simulink model "sedemo_discouragearrival"  (Simulink 7.5)
settings: Solver=VariableStepDiscrete  StartTime=0.0  StopTime=100000  MaxStep=inf  RelTol=1e-3
PostLoadFcn:
  | open_system([gcs '/Service Rate Gain']);
  | open_system([gcs '/Waiting Time Comparison:  Theory vs. Simulation']);
undefined symbols (not defined in the file or in its folder): des_subsystemblock, des_subsysteminport, des_subsystemoutport, des_subsystemsupportblock
libraries: simulink x2, simeventstranslate1 x2, simeventssink1 x1, simeventsqueue1 x1, simeventsinfo x1, simeventsserver1 x1, simeventsgenerators1 x1
CloseFcn:
  | close_system([gcs '/Service Rate Gain']);
  | close_system([gcs '/Waiting Time Comparison:  Theory vs. Simulation']);
settings Model: Creator=The MathWorks Inc.  ExtModeAutoUpdateStatusClock=off
settings DataIOCC: SaveOutput=off  SaveTime=off
settings OptimizationCC: InlineInvariantSignals=on  InitFltsAndDblsToZero=on  BufferReusableBoundary=off
settings DebuggingCC: AlgebraicLoopMsg=error  SaveWithParameterizedLinksMsg=none  SignalResolutionControl=TryResolveAllWithWarning  SolverPrmCheckMsg=none  MultiTaskDSMMsg=warning  MultiTaskCondExecSysMsg=none  SigSpecEnsureSampleTimeMsg=none  BusObjectLabelMismatch=none  StrictBusMsg=None
settings RTWCC: IncludeERTFirstTime=on
settings GRTTargetCC: TargetFcnLib=ansi_tfl_tmw.mat
settings SimEventsCC: propIdentEventSeed=12345678  propDiagAttribOutput=1  propDiagFcnCallOutput=1  propDiagStatOutput=0

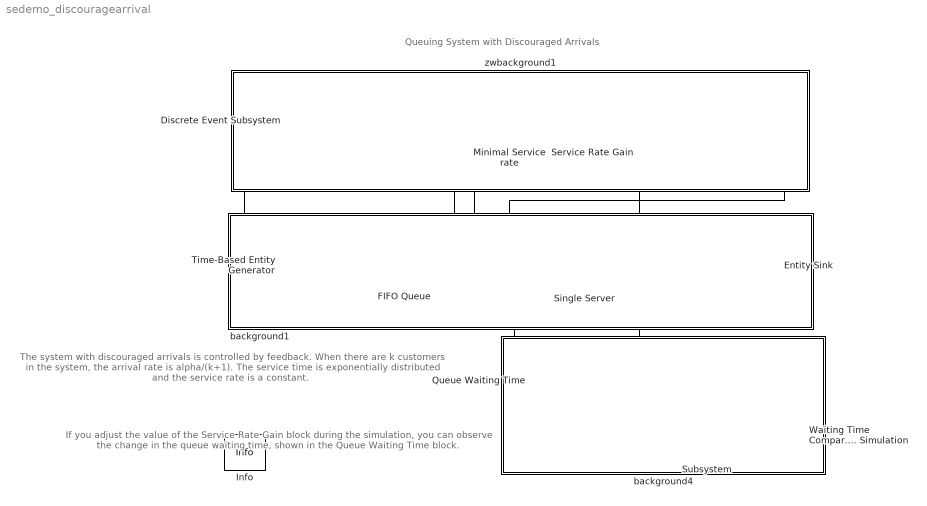
== system sedemo_discouragearrival ==
  note: Queuing System with Discouraged Arrivals
  note: The system with discouraged arrivals is
      | controlled by feedback. When there are k
      | customers in the system, the arrival rate is
      | alpha/(k+1). The service time is exponentially
      | distributed and the service rate is a constant.
  note: If you adjust the value of the Service Rate
      | Gain block during the simulation, you
      | can observe the change in the queue waiting
      | time, shown in the Queue Waiting Time block.
  "  " : Subsystem  mask(Exponential Service Time Distribution){seed=1234567}
      mask prompts: seed "Initial seed"
      mask help: For a given input service rate, output an exponentially distributed random number. Output is repeatable for a given seed.
      mask Display: disp('Exponential\nService Time\nDistribution');
  Discrete Event Subsystem : Subsystem  LoadFcn=des_subsystemblock(gcb, 'load');  InitFcn=des_subsystemblock(gcb, 'init');  StartFcn=des_subsystemblock(gcb, 'start');  StopFcn=des_subsystemblock(gcb, 'stop');  mask(Discrete Event Subsystem){seed=9876543}
      mask prompts: seed "Initial seed:"
      settings: CopyFcn=des_subsystemblock(gcb, 'copy');  DeleteFcn=des_subsystemblock(gcb, 'delete');  UndoDeleteFcn=des_subsystemblock(gcb, 'undodelete');  ModelCloseFcn=des_subsystemblock(gcb, 'modelclose');  PreSaveFcn=des_subsystemblock(gcb, 'presave');  NameChangeFcn=des_subsystemblock(gcb, 'namechange');  OpenFcn=des_subsystemblock(gcb, 'open');  ParentCloseFcn=des_subsystemblock(gcb, 'parentclose');  ErrorFcn=des_subsystemerror
      mask Help: helpview(simeventsbhelp);
      mask Display: disp('Interarrival Time Distribution\n with Discouraged Rate\n(Alpha=1)');
  Entity Sink : simeventssink1/Entity Sink  Priority=1  SystemSampleTime=-1  AvailableForArrivals=on  StatNumberArrived=Off
  FIFO Queue : simeventsqueue1/FIFO Queue  Priority=1  SystemSampleTime=-1  Capacity=Inf  EnableTOPort=off  StatNumberDeparted=Off  StatNumberInBlock=On  StatPendingEntity=Off  StatAverageWait=On  StatAverageQueueLength=Off  StatNumberTimedout=Off
  Info : simeventsinfo/Info  SystemSampleTime=-1
  Minimal Service rate : Constant  OutDataType=sfix(16)  OutScaling=2^0
  Queue Waiting Time : Display
  Service Rate Gain : simulink/Math Operations/Slider Gain  SystemSampleTime=-1  low=0.1  gain=3  high=10
  Single Server : simeventsserver1/Single Server  Priority=1  SystemSampleTime=-1  ServiceTimeFrom=Signal port t  ServiceTime=1  AttributeName=ServiceTime  PriorityServiceCompletion=1  PermitPreemption=off  SortingAttributeName=PriorityAttributeName  SortingDirection=Ascending  WriteToAttribute=off  ResidualAttributeName=ResidualServiceTime  CreateAttribute=on  EnableTOPort=off  StatNumberDeparted=Off  StatNumberInBlock=On  StatNumberPreempted=Off  StatPendingEntity=Off  StatAverageWait=Off  StatUtilization=Off  StatNumberTimedout=Off
  Subsystem : Subsystem
      mask Type: Waiting Time Evaluation for Discouraged Arrivals
      mask Description: For a given input service rate and alpha=1, evaluate waiting time for discouraged arrivals. Combine and output the theoretical and simulation results.
      mask Display: disp('Waiting Time\nEvaluation');
  Time-Based Entity Generator : simeventsgenerators1/Entity Generators/Time-Based Entity Generator  Priority=1  DialogController=des_ddg_create  DialogControllerArgs=DataTag13  SystemSampleTime=-1  GenerateEntitiesUpon=Intergeneration time from port t  Distribution=Constant  Minimum=0  Maximum=1  Mean=1  InitialSeed=12345  Period=1  PriorityEntityGeneration=1  GenerateEntityAtSimulationStart=on  ResponseWhenBlocked=Pause generation  ResponseWhenUnblocked=Immediate restart  EntityType=Standard  StatNumberDeparted=Off  StatPendingEntity=Off  StatAverageIntergenerationTime=Off
  Waiting Time Comparison:  Theory vs. Simulation : Scope
      settings: YMin=0  YMax=0.15
  background1 : Subsystem
      mask Display: disp('')
  background4 : Subsystem
      mask Display: disp('')
  zwbackground1 : Subsystem
      mask Display: disp('')
  wires:
  "  "/1(Out1) -> Single Server/1
  Discrete Event Subsystem/1(Dout) -> Time-Based Entity Generator/1
  Single Server/1 -> Discrete Event Subsystem/1(Din)
  Minimal Service rate/1 -> Service Rate Gain/1
  Service Rate Gain/1 -> "  "/1(Service rate), Subsystem/1(mu)
  Subsystem/1(Out1) -> Waiting Time Comparison:  Theory vs. Simulation/1
  FIFO Queue/1 -> Discrete Event Subsystem/2(Din1)
  FIFO Queue/2 -> Queue Waiting Time/1, Subsystem/2(waiting time measurement)
  connections:
  Time-Based Entity Generator/RConn1 -- FIFO Queue/LConn1
  FIFO Queue/RConn1 -- Single Server/LConn1
  Single Server/RConn1 -- Entity Sink/LConn1

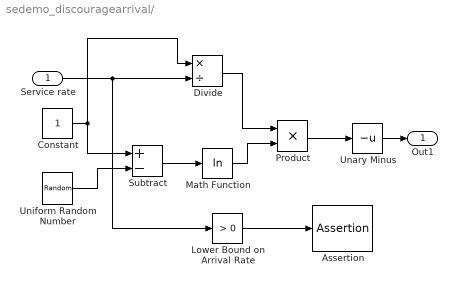
== system sedemo_discouragearrival/   ==
  Service rate : Inport  OutDataType=sfix(16)  OutScaling=2^0
  Assertion : Assertion  Enabled=on
  Constant : Constant  OutDataType=sfix(16)  OutScaling=2^0
  Divide : Product  Inputs=*/  OutDataType=sfix(16)  OutScaling=2^-10
  Lower Bound on Arrival Rate : simulink/Logic and Bit Operations/Compare To Constant  SystemSampleTime=-1  relop=>  const=0  LogicOutDataTypeMode=uint8  ZeroCross=off
  Math Function : Math  Operator=log  OutDataType=sfix(16)  OutScaling=2^0  SaturateOnIntegerOverflow=on
  Product : Product  OutDataType=sfix(16)  OutScaling=2^0  RndMeth=Zero
  Subtract : Sum  Inputs=+-  OutDataType=sfix(16)  OutScaling=2^-10
  Unary Minus : UnaryMinus
  Uniform Random Number : UniformRandomNumber  Minimum=0  Seed=seed  SampleTime=0
  Out1 : Outport  OutDataType=sfix(16)  OutScaling=2^0
  wires:
  Unary Minus/1 -> Out1/1
  Product/1 -> Unary Minus/1
  Math Function/1 -> Product/2
  Subtract/1 -> Math Function/1
  Uniform Random Number/1 -> Subtract/2
  Constant/1 -> Subtract/1, Divide/1
  Service rate/1 -> Divide/2, Lower Bound on Arrival Rate/1
  Divide/1 -> Product/1
  Lower Bound on Arrival Rate/1 -> Assertion/1

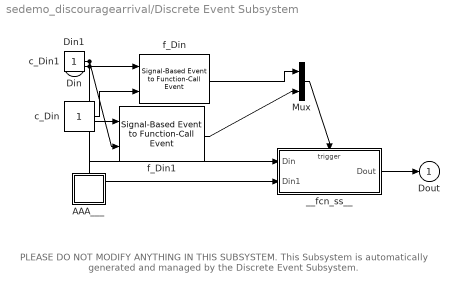
== system sedemo_discouragearrival/Discrete Event Subsystem ==
  note: PLEASE DO NOT MODIFY ANYTHING IN THIS SUBSYSTEM.
      | This Subsystem is automatically generated and
      | managed by the Discrete Event Subsystem.
  Din : Inport  PortDimensions=1  DataType=double  OutDataType=sfix(16)  OutScaling=2^0  OutDataTypeStr=double
  Din1 : Inport  Port=2  PortDimensions=1  DataType=double  OutDataType=sfix(16)  OutScaling=2^0  OutDataTypeStr=double
  AAA___ : Subsystem  LoadFcn=des_subsystemsupportblock(gcb, 'load');  InitFcn=des_subsystemsupportblock(gcb, 'init');  StartFcn=des_subsystemsupportblock(gcb, 'start');  StopFcn=des_subsystemsupportblock(gcb, 'stop');
      settings: CopyFcn=des_subsystemsupportblock(gcb, 'copy');  DeleteFcn=des_subsystemsupportblock(gcb, 'delete');  UndoDeleteFcn=des_subsystemsupportblock(gcb, 'undodelete');  ModelCloseFcn=des_subsystemsupportblock(gcb, 'modelclose');  PreSaveFcn=des_subsystemsupportblock(gcb, 'presave');  NameChangeFcn=des_subsystemsupportblock(gcb, 'namechange');  OpenFcn=des_subsystemsupportblock(gcb, 'open');  ParentCloseFcn=des_subsystemsupportblock(gcb, 'parentclose');
  Mux : Mux  Inputs=2
  __fcn_ss__ : Subsystem  TreatAsAtomicUnit=on
      settings: PropExecContextOutsideSubsystem=on
  c_Din : Constant  OutDataType=sfix(16)  OutScaling=2^0
  c_Din1 : Constant  OutDataType=sfix(16)  OutScaling=2^0
  f_Din : simeventstranslate1/Signal-Based Event to Function-Call Event  Priority=1  SystemSampleTime=-1  GenerateFunctionCallUpon=Sample time hit from port ts  SignalEdgeOption=Rising  EnableE1Port=on  EnableF2Port=off  EnableE2Port=off  SpecifyEventPriority=off  PriorityFunctionCall=20  FunctionCallDelayFrom=Dialog  DelayFunctionCall=0  StatNumberF1Calls=Off  StatNumberF2Calls=Off  MaskBlockType=none
  f_Din1 : simeventstranslate1/Signal-Based Event to Function-Call Event  Priority=1  SystemSampleTime=-1  GenerateFunctionCallUpon=Sample time hit from port ts  SignalEdgeOption=Rising  EnableE1Port=on  EnableF2Port=off  EnableE2Port=off  SpecifyEventPriority=off  PriorityFunctionCall=20  FunctionCallDelayFrom=Dialog  DelayFunctionCall=0  StatNumberF1Calls=Off  StatNumberF2Calls=Off  MaskBlockType=none
  Dout : Outport  OutDataType=sfix(16)  OutScaling=2^0
  wires:
  __fcn_ss__/1(Dout) -> Dout/1
  f_Din/1 -> Mux/1
  c_Din/1 -> f_Din/2
  Mux/1 -> __fcn_ss__/Trigger
  f_Din1/1 -> Mux/2
  c_Din1/1 -> f_Din1/2
  Din/1 -> f_Din/1, __fcn_ss__/1(Din)
  Din1/1 -> f_Din1/1, __fcn_ss__/2(Din1)

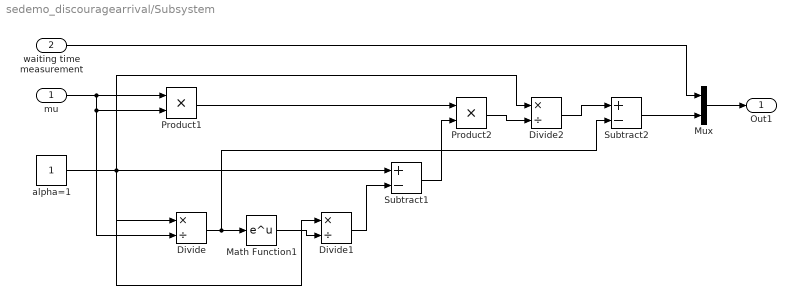
== system sedemo_discouragearrival/Subsystem ==
  mu : Inport  OutDataType=sfix(16)  OutScaling=2^0
  waiting time measurement : Inport  Port=2  OutDataType=sfix(16)  OutScaling=2^0
  Divide : Product  Inputs=*/  OutDataType=sfix(16)  OutScaling=2^-10
  Divide1 : Product  Inputs=*/  OutDataType=sfix(16)  OutScaling=2^-10
  Divide2 : Product  Inputs=*/  OutDataType=sfix(16)  OutScaling=2^-10
  Math Function1 : Math  OutDataType=sfix(16)  OutScaling=2^0  SaturateOnIntegerOverflow=on
  Mux : Mux  Inputs=2
  Product1 : Product  OutDataType=sfix(16)  OutScaling=2^0  RndMeth=Zero
  Product2 : Product  OutDataType=sfix(16)  OutScaling=2^0  RndMeth=Zero
  Subtract1 : Sum  Inputs=+-  OutDataType=sfix(16)  OutScaling=2^-10
  Subtract2 : Sum  Inputs=+-  OutDataType=sfix(16)  OutScaling=2^-10
  alpha=1 : Constant  OutDataType=sfix(16)  OutScaling=2^0
  Out1 : Outport  OutDataType=sfix(16)  OutScaling=2^0
  wires:
  mu/1 -> Divide/2, Product1/2, Product1/1
  alpha=1/1 -> Subtract1/1, Divide/1, Divide1/1, Divide2/1
  Divide/1 -> Math Function1/1, Subtract2/2
  Math Function1/1 -> Divide1/2
  Divide1/1 -> Subtract1/2
  Product1/1 -> Product2/1
  Subtract1/1 -> Product2/2
  Product2/1 -> Divide2/2
  waiting time measurement/1 -> Mux/1
  Mux/1 -> Out1/1
  Divide2/1 -> Subtract2/1
  Subtract2/1 -> Mux/2

== system sedemo_discouragearrival/background1 ==

== system sedemo_discouragearrival/background4 ==

== system sedemo_discouragearrival/zwbackground1 ==
  note: This subsystem is empty

== system sedemo_discouragearrival/Discrete Event Subsystem/AAA___ ==

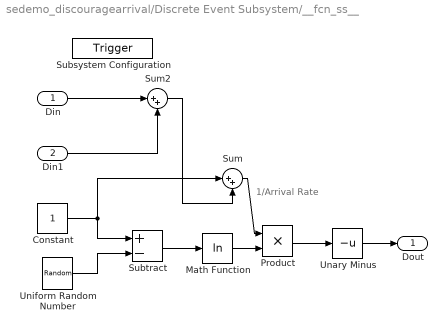
== system sedemo_discouragearrival/Discrete Event Subsystem/__fcn_ss__ ==
  note: 1/Arrival Rate
  Din : Inport  LoadFcn=des_subsysteminport(gcb, 'load');  InitFcn=des_subsysteminport(gcb, 'init');  StartFcn=des_subsysteminport(gcb, 'start');  StopFcn=des_subsysteminport(gcb, 'stop');  OutDataType=sfix(16)  OutScaling=2^0  mask(Discrete Event Inport){PermitSubsystemEvents=on, TypeOfEvent=Sample time hit, SignalEdgeOption=Rising, SpecifyEventPriority=off, PrioritySubsystemEvent=20}
      mask prompts: PermitSubsystemEvents "Execute subsystem upon signal-based events"; TypeOfEvent "Type of signal-based event:"; SignalEdgeOption "Type of change in signal value:"; SpecifyEventPriority "Specify event priority for executing subsystem"; PrioritySubsystemEvent "Subsystem execution event priority:"
      mask help: Input port for a Discrete Event Subsystem block. This block can conditionally execute the subsystem upon signal-based events that meet specified criteria.
      mask init:
      | des_subsystemmask(gcb, 'init','apply')
      settings: CopyFcn=des_subsysteminport(gcb, 'copy');  DeleteFcn=des_subsysteminport(gcb, 'delete');  UndoDeleteFcn=des_subsysteminport(gcb, 'undodelete');  ModelCloseFcn=des_subsysteminport(gcb, 'modelclose');  PreSaveFcn=des_subsysteminport(gcb, 'presave');  NameChangeFcn=des_subsysteminport(gcb, 'namechange');  ParentCloseFcn=des_subsysteminport(gcb, 'parentclose');
      mask Help: helpview(simeventsbhelp);
      mask StyleString: checkbox,popup(Change in signal|Trigger|Sample time hit),popup(Rising|Falling|Either),checkbox,edit
      mask CallbackString: des_subsystemmask(gcb, 'cbPermitSubsystemEvents', 'noapply');|des_subsystemmask(gcb,'cbTypeOfEvent','noapply');||des_subsystemmask(gcb, 'cbSpecifyEventPriority', 'noapply');|
  Din1 : Inport  LoadFcn=des_subsysteminport(gcb, 'load');  InitFcn=des_subsysteminport(gcb, 'init');  StartFcn=des_subsysteminport(gcb, 'start');  StopFcn=des_subsysteminport(gcb, 'stop');  Port=2  OutDataType=sfix(16)  OutScaling=2^0  mask(Discrete Event Inport){PermitSubsystemEvents=on, TypeOfEvent=Sample time hit, SignalEdgeOption=Rising, SpecifyEventPriority=off, PrioritySubsystemEvent=20}
      mask prompts: PermitSubsystemEvents "Execute subsystem upon signal-based events"; TypeOfEvent "Type of signal-based event:"; SignalEdgeOption "Type of change in signal value:"; SpecifyEventPriority "Specify event priority for executing subsystem"; PrioritySubsystemEvent "Subsystem execution event priority:"
      mask help: Input port for a Discrete Event Subsystem block. This block can conditionally execute the subsystem upon signal-based events that meet specified criteria.
      mask init:
      | des_subsystemmask(gcb, 'init','apply')
      settings: CopyFcn=des_subsysteminport(gcb, 'copy');  DeleteFcn=des_subsysteminport(gcb, 'delete');  UndoDeleteFcn=des_subsysteminport(gcb, 'undodelete');  ModelCloseFcn=des_subsysteminport(gcb, 'modelclose');  PreSaveFcn=des_subsysteminport(gcb, 'presave');  NameChangeFcn=des_subsysteminport(gcb, 'namechange');  ParentCloseFcn=des_subsysteminport(gcb, 'parentclose');
      mask Help: helpview(simeventsbhelp);
      mask StyleString: checkbox,popup(Change in signal|Trigger|Sample time hit),popup(Rising|Falling|Either),checkbox,edit
      mask CallbackString: des_subsystemmask(gcb, 'cbPermitSubsystemEvents', 'noapply');|des_subsystemmask(gcb,'cbTypeOfEvent','noapply');||des_subsystemmask(gcb, 'cbSpecifyEventPriority', 'noapply');|
  Subsystem Configuration : TriggerPort  TriggerType=function-call
      settings: CopyFcn=des_subsystemconfigblock(gcb, 'copy');  DeleteFcn=des_subsystemconfigblock(gcb, 'delete');  UndoDeleteFcn=des_subsystemconfigblock(gcb, 'undodelete');
      mask Type: Subsystem Configuration
      mask Description: Configuration for a Discrete Event Subsystem block. Every discrete event subsystem window must contain exactly one copy of this configuration block. Do not delete this block.
      mask Help: helpview(simeventsbhelp);
      mask Display: disp('Do Not Delete');
  Constant : Constant  OutDataType=sfix(16)  OutScaling=2^0
  Math Function : Math  Operator=log  OutDataType=sfix(16)  OutScaling=2^0  SaturateOnIntegerOverflow=on
  Product : Product  OutDataType=sfix(16)  OutScaling=2^0  RndMeth=Zero
  Subtract : Sum  Inputs=+-  OutDataType=sfix(16)  OutScaling=2^-10
  Sum : Sum  Inputs=|++  OutDataType=sfix(16)  OutScaling=2^0
  Sum2 : Sum  Inputs=|++  OutDataType=sfix(16)  OutScaling=2^0
  Unary Minus : UnaryMinus
  Uniform Random Number : UniformRandomNumber  Minimum=0  Seed=seed
  Dout : Outport  LoadFcn=des_subsystemoutport(gcb, 'load');  InitFcn=des_subsystemoutport(gcb, 'init');  StartFcn=des_subsystemoutport(gcb, 'start');  StopFcn=des_subsystemoutport(gcb, 'stop');  OutDataType=sfix(16)  OutScaling=2^0
      settings: CopyFcn=des_subsystemoutport(gcb, 'copy');  DeleteFcn=des_subsystemoutport(gcb, 'delete');  UndoDeleteFcn=des_subsystemoutport(gcb, 'undodelete');  ModelCloseFcn=des_subsystemoutport(gcb, 'modelclose');  PreSaveFcn=des_subsystemoutport(gcb, 'presave');  NameChangeFcn=des_subsystemoutport(gcb, 'namechange');  ParentCloseFcn=des_subsystemoutport(gcb, 'parentclose');
      mask Type: Discrete Event Outport
      mask Description: Provide an output port for a Discrete Event Subsystem block.
      mask Help: helpview(simeventsbhelp);
  wires:
  Product/1 -> Unary Minus/1
  Math Function/1 -> Product/2
  Subtract/1 -> Math Function/1
  Uniform Random Number/1 -> Subtract/2
  Constant/1 -> Subtract/1, Sum/1
  Sum2/1 -> Sum/2
  Sum/1 -> Product/1
  Din/1 -> Sum2/1
  Din1/1 -> Sum2/2
  Unary Minus/1 -> Dout/1
